simulink model "softarm_constrained_plant"  (R2025a)
settings: Solver=ode15s  StartTime=0.0  StopTime=5  RelTol=1e-3
model mask{Bundle=Bundle}
  mask prompts: Bundle "Bundle directory"
PreLoadFcn:
  | softarm_root=fileparts(get_param(bdroot,'FileName'));addpath(softarm_root);addpath(fullfile(softarm_root,'matlab'));
model workspace (MAT data in the model file):
  Bundle = 'examples/generated/pcc_flying_plane_contact_n1'
undefined symbols (not defined in the file or in its folder): softarm_nq, softarm_p, softarm_x0
settings Model: ParameterArgumentNames=Bundle  Creator=rlwan  LastModifiedBy=rlwan

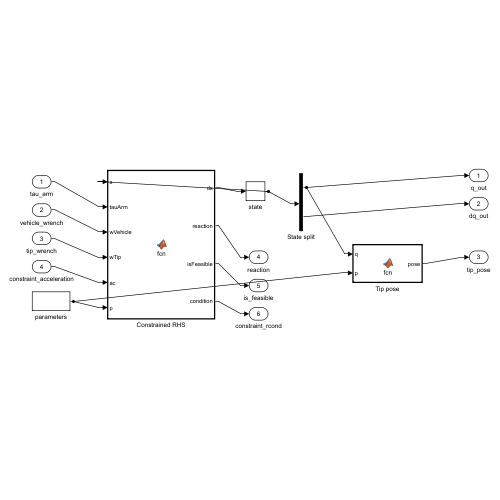
[thumbnail: Simulink's stored preview of the top-level diagram]
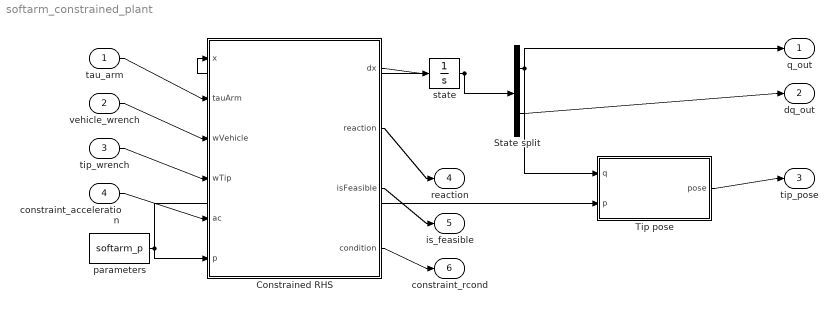
== system softarm_constrained_plant ==
  tau_arm : Inport  PortDimensions=softarm_narm
  vehicle_wrench : Inport  Port=2  PortDimensions=6
  tip_wrench : Inport  Port=3  PortDimensions=6
  constraint_acceleration : Inport  Port=4  PortDimensions=softarm_nc
  Constrained RHS : MATLAB Function  TreatAsAtomicUnit=on
  State split : Demux  Outputs=[softarm_nq softarm_nq]
  Tip pose : MATLAB Function  TreatAsAtomicUnit=on
  parameters : Constant  Value=softarm_p
  state : Integrator  InitialCondition=softarm_x0
  q_out : Outport
  dq_out : Outport  Port=2
  tip_pose : Outport  Port=3
  reaction : Outport  Port=4
  is_feasible : Outport  Port=5
  constraint_rcond : Outport  Port=6
  wires:
  state/1 -> State split/1, Constrained RHS/1(x)
  tau_arm/1 -> Constrained RHS/2(tauArm)
  vehicle_wrench/1 -> Constrained RHS/3(wVehicle)
  tip_wrench/1 -> Constrained RHS/4(wTip)
  constraint_acceleration/1 -> Constrained RHS/5(ac)
  parameters/1 -> Constrained RHS/6(p), Tip pose/2(p)
  Constrained RHS/1(dx) -> state/1
  Constrained RHS/2(reaction) -> reaction/1
  Constrained RHS/3(isFeasible) -> is_feasible/1
  Constrained RHS/4(condition) -> constraint_rcond/1
  State split/1 -> q_out/1, Tip pose/1(q)
  State split/2 -> dq_out/1
  Tip pose/1(pose) -> tip_pose/1

== matlab function softarm_constrained_plant/Tip pose ==
  data: q input; pose output; p input
function pose = fcn(q,p)
%#codegen
H=softarm_kinematics(q,p); pose=reshape(H(:,:,end),16,1);
end

== matlab function softarm_constrained_plant/Constrained RHS ==
  data: x input; dx output; tauArm input; wVehicle input; wTip input; ac input; p input; reaction output; isFeasible output; condition output
function [dx,reaction,isFeasible,condition] = fcn(x,tauArm,wVehicle,wTip,ac,p)
%#codegen
n=numel(x)/2; q=x(1:n); dq=x(n+1:end);
[ddq,reaction,isFeasible,condition]=softarm_constraint_acceleration(q,dq,tauArm,wVehicle,wTip,ac,p);
dx=[dq;ddq];
end
